simulink model "grandland_sim"  (R2022b)
settings: Solver=VariableStepAuto  StartTime=0.0  StopTime=10.0  RelTol=1e-3
values from neighbouring files (symbols this model uses):
  r = 0.033    [grandland.m]    (also in grandland_3.m; test.m)
libraries: cstblocks x4
settings Model: Creator=antor  LastModifiedBy=antor

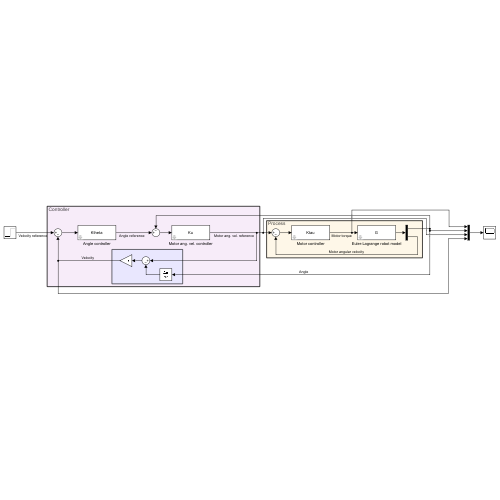
[thumbnail: Simulink's stored preview of the top-level diagram]
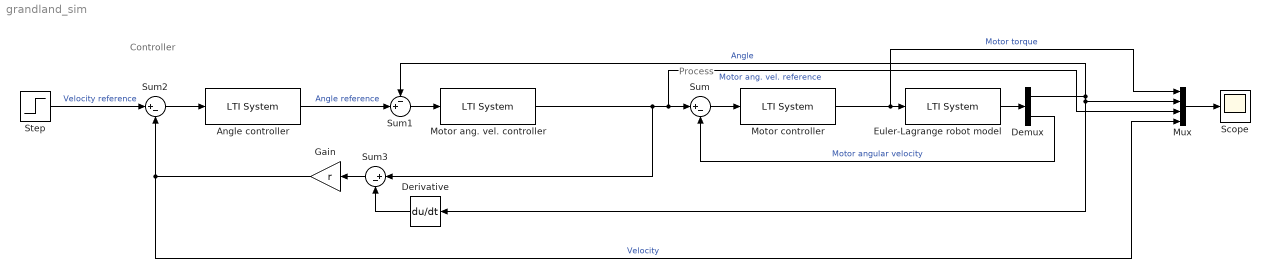
== system grandland_sim ==
  note: Controller
  note: Process
  Angle controller : cstblocks/LTI System  sys=Ktheta  IC=[]
  Demux : Demux  Outputs=2
  Derivative : Derivative
  Euler-Lagrange robot model : cstblocks/LTI System  sys=G  IC=[]
  Gain : Gain  Gain=r
  Motor ang. vel. controller : cstblocks/LTI System  sys=Ku  IC=[]
  Motor controller : cstblocks/LTI System  sys=Ktau  IC=[]
  Mux : Mux
  Scope : Scope
  Step : Step  After=0.1  SampleTime=0
  Sum : Sum  Inputs=|+-
  Sum1 : Sum  Inputs=-+|
  Sum2 : Sum  Inputs=|+-
  Sum3 : Sum  Inputs=|+-
  wires:
  Motor controller/1 -> Mux/1, Euler-Lagrange robot model/1  "Motor torque"
  Euler-Lagrange robot model/1 -> Demux/1
  Demux/2 -> Sum/2  "Motor angular velocity"
  Sum/1 -> Motor controller/1
  Motor ang. vel. controller/1 -> Sum3/1, Mux/3, Sum/1  "Motor ang. vel. reference"
  Sum1/1 -> Motor ang. vel. controller/1
  Demux/1 -> Mux/2, Derivative/1, Sum1/1  "Angle"
  Angle controller/1 -> Sum1/2  "Angle reference"
  Sum2/1 -> Angle controller/1
  Derivative/1 -> Sum3/2
  Sum3/1 -> Gain/1
  Gain/1 -> Mux/4, Sum2/2  "Velocity"
  Step/1 -> Sum2/1  "Velocity reference"
  Mux/1 -> Scope/1
